simulink model "vector_sin_controller_test"  (R2023a)
settings: Solver=FixedStepAuto  StartTime=0.0  StopTime=10.0  FixedStep=0.0001  RelTol=1e-3
settings Model: Creator=motya  LastModifiedBy=motya

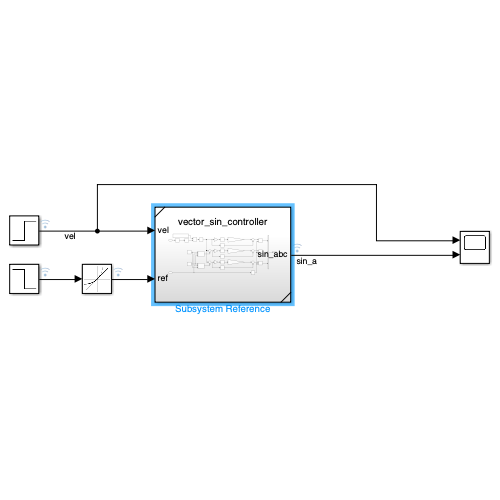
[thumbnail: Simulink's stored preview of the top-level diagram]
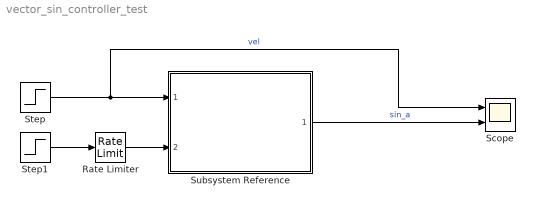
== system vector_sin_controller_test ==
  Rate Limiter : RateLimiter  SampleTimeMode=inherited
  Scope : Scope  NumInputPorts=2
  Step : Step  Time=2  Before=1  After=2  SampleTime=0
  Step1 : Step  Time=5  Before=1  After=-2  SampleTime=0
  Subsystem Reference : Subsystem  ReferencedSubsystem=vector_sin_controller
  wires:
  Step/1 -> Scope/1, Subsystem Reference/1  "vel"
  Step1/1 -> Rate Limiter/1
  Subsystem Reference/1 -> Scope/2  "sin_a"
  Rate Limiter/1 -> Subsystem Reference/2
